simulink model "E3"  (R2014a)
settings: Solver=ode45  StartTime=0.0  StopTime=30  RelTol=1e-3
values from neighbouring files (symbols this model uses):
  Kc = 1    [E01.m]
  Kr = 1    [E01.m]
  s = tf('s')    [E01.m]
libraries: cstblocks x2, simulink x1
settings Model: Creator=Davide  LastModifiedBy=Davide

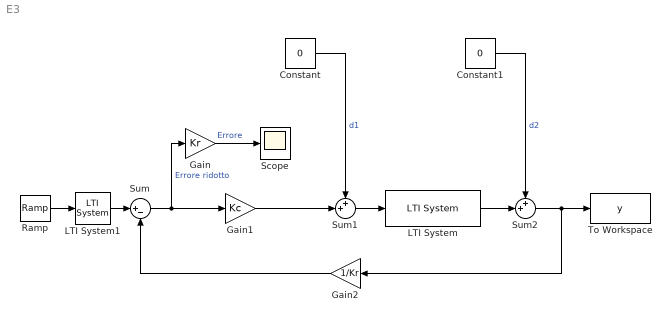
== system E3 ==
  Constant : Constant  Value=0
  Constant1 : Constant  Value=0
  Gain : Gain  Gain=Kr
  Gain1 : Gain  Gain=Kc
  Gain2 : Gain  Gain=1/Kr
  LTI System : cstblocks/LTI System  sys=F  IC=[]
  LTI System1 : cstblocks/LTI System  sys=1/s  IC=[]
  Ramp : simulink/Sources/Ramp  slope=1  start=0  X0=0
  Scope : Scope
  Sum : Sum  Inputs=|+-
  Sum1 : Sum  Inputs=++|
  Sum2 : Sum  Inputs=++|
  To Workspace : ToWorkspace  VariableName=y  SaveFormat=Timeseries  SampleTime=-1
  wires:
  Ramp/1 -> LTI System1/1
  Constant/1 -> Sum1/1  "d1"
  Sum/1 -> Gain/1, Gain1/1  "Errore ridotto"
  Sum1/1 -> LTI System/1
  LTI System/1 -> Sum2/2
  Constant1/1 -> Sum2/1  "d2"
  Sum2/1 -> Gain2/1, To Workspace/1
  Gain/1 -> Scope/1  "Errore"
  Gain1/1 -> Sum1/2
  Gain2/1 -> Sum/2
  LTI System1/1 -> Sum/1
